simulink model "Prac02_2_2"  (R2015a)
settings: Solver=ode45  StartTime=0.0  StopTime=8.0  RelTol=1e-3
libraries: dsparch4 x3
settings Model: Creator=redes  LastModifiedBy=Josemi

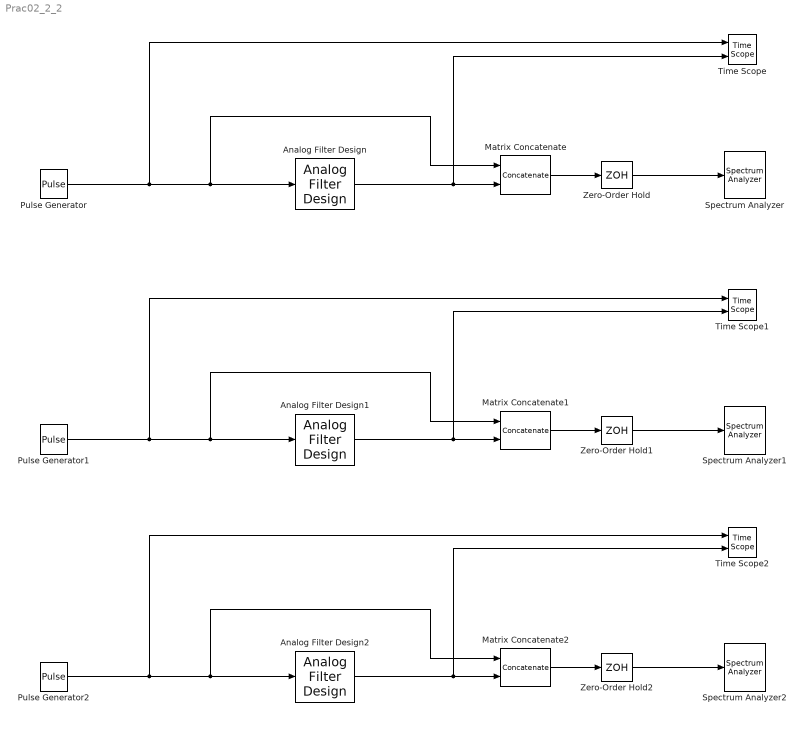
== system Prac02_2_2 ==
  Analog Filter Design : dsparch4/Analog Filter Design  method=Chebyshev II  filttype=Lowpass  N=8  Wlo=2*pi*20  Whi=80  Rp=2  Rs=20
  Analog Filter Design1 : dsparch4/Analog Filter Design  method=Chebyshev II  filttype=Lowpass  N=8  Wlo=2*pi*80  Whi=80  Rp=2  Rs=20
  Analog Filter Design2 : dsparch4/Analog Filter Design  method=Chebyshev II  filttype=Lowpass  N=8  Wlo=2*pi*80  Whi=80  Rp=2  Rs=20
  Matrix Concatenate : Concatenate  Mode=Multidimensional array  ConcatenateDimension=2
  Matrix Concatenate1 : Concatenate  Mode=Multidimensional array  ConcatenateDimension=2
  Matrix Concatenate2 : Concatenate  Mode=Multidimensional array  ConcatenateDimension=2
  Pulse Generator : DiscretePulseGenerator  PulseType=Time based  Period=1  PulseWidth=50
  Pulse Generator1 : DiscretePulseGenerator  PulseType=Time based  Period=0.25  PulseWidth=50
  Pulse Generator2 : DiscretePulseGenerator  PulseType=Time based  Period=1  PulseWidth=50
  Spectrum Analyzer : SpectrumAnalyzer
  Spectrum Analyzer1 : SpectrumAnalyzer
  Spectrum Analyzer2 : SpectrumAnalyzer
  Time Scope : TimeScope  DefaultConfigurationName=spbscopes.TimeScopeBlockCfg  NumInputPorts=2
  Time Scope1 : TimeScope  DefaultConfigurationName=spbscopes.TimeScopeBlockCfg  NumInputPorts=2
  Time Scope2 : TimeScope  DefaultConfigurationName=spbscopes.TimeScopeBlockCfg  NumInputPorts=2
  Zero-Order Hold : ZeroOrderHold  SampleTime=0.0025
  Zero-Order Hold1 : ZeroOrderHold  SampleTime=0.0025
  Zero-Order Hold2 : ZeroOrderHold  SampleTime=0.0025
  wires:
  Pulse Generator/1 -> Time Scope/1, Matrix Concatenate/1, Analog Filter Design/1
  Analog Filter Design/1 -> Time Scope/2, Matrix Concatenate/2
  Matrix Concatenate/1 -> Zero-Order Hold/1
  Zero-Order Hold/1 -> Spectrum Analyzer/1
  Pulse Generator1/1 -> Time Scope1/1, Matrix Concatenate1/1, Analog Filter Design1/1
  Analog Filter Design1/1 -> Time Scope1/2, Matrix Concatenate1/2
  Matrix Concatenate1/1 -> Zero-Order Hold1/1
  Zero-Order Hold1/1 -> Spectrum Analyzer1/1
  Pulse Generator2/1 -> Time Scope2/1, Matrix Concatenate2/1, Analog Filter Design2/1
  Analog Filter Design2/1 -> Time Scope2/2, Matrix Concatenate2/2
  Matrix Concatenate2/1 -> Zero-Order Hold2/1
  Zero-Order Hold2/1 -> Spectrum Analyzer2/1
